simulink subsystem "PID_maneuver"  (R2021a)
settings: Solver=VariableStepAuto  StartTime=0.0  StopTime=10.0  RelTol=1e-3
undefined symbols (not defined in the file): Tmax
libraries: vrlib x1
settings Model: Creator=Laura  LastModifiedBy=Laura

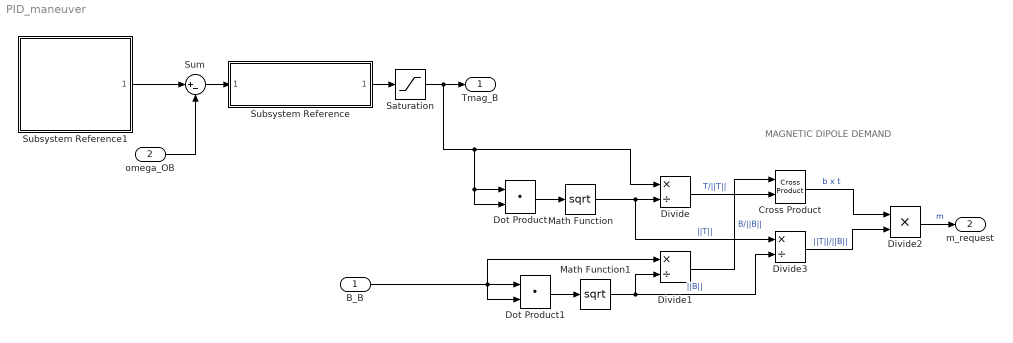
== system PID_maneuver ==
  note: MAGNETIC DIPOLE DEMAND
  B_B : Inport
  "omega_OB " : Inport  Port=2
  Cross Product : vrlib/Utilities/Cross Product
  Divide : Product  Inputs=*/
  Divide1 : Product  Inputs=*/
  Divide2 : Product  Inputs=**
  Divide3 : Product  Inputs=*/
  Dot Product : DotProduct  InputSameDT=on  OutDataTypeStr=Inherit: Inherit via internal rule
  Dot Product1 : DotProduct  InputSameDT=on  OutDataTypeStr=Inherit: Inherit via internal rule
  Math Function : Math  Operator=sqrt  SignedPower=on  SaturateOnIntegerOverflow=on
  Math Function1 : Math  Operator=sqrt  SignedPower=on  SaturateOnIntegerOverflow=on
  Saturation : Saturate  UpperLimit=Tmax  LowerLimit=-Tmax
  Subsystem Reference : Subsystem  ReferencedSubsystem=PID
  Subsystem Reference1 : Subsystem  ReferencedSubsystem=Maneuver
  Sum : Sum  Inputs=|+-
  Tmag_B : Outport
  m_request : Outport  Port=2
  wires:
  Subsystem Reference1/1 -> Sum/1
  "omega_OB "/1 -> Sum/2
  Sum/1 -> Subsystem Reference/1
  Saturation/1 -> Dot Product/2, Dot Product/1, Divide/1, Tmag_B/1
  Dot Product/1 -> Math Function/1
  Dot Product1/1 -> Math Function1/1
  B_B/1 -> Dot Product1/1, Dot Product1/2, Divide1/1
  Math Function/1 -> Divide/2, Divide3/1  "||T||"
  Math Function1/1 -> Divide3/2, Divide1/2  "||B||"
  Divide/1 -> Cross Product/2  "T/||T||"
  Divide1/1 -> Cross Product/1  "B/||B||"
  Cross Product/1 -> Divide2/1  "b x t"
  Divide3/1 -> Divide2/2  "||T||/||B||"
  Divide2/1 -> m_request/1  "m"
  Subsystem Reference/1 -> Saturation/1
